simulink model "test_sim"  (R2020b)
settings: Solver=VariableStepAuto  StartTime=0.0  StopTime=10.0  RelTol=1e-3
libraries: fuzblock x1
settings Model: Creator=lima  LastModifiedBy=lima

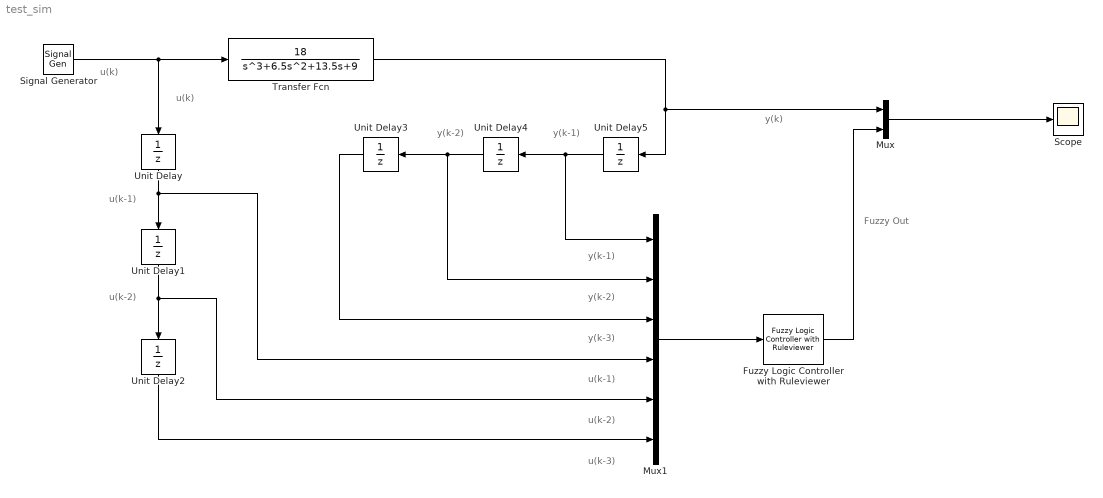
== system test_sim ==
  note: u(k)
  note: u(k-3)
  note: u(k-2)
  note: u(k-1)
  note: y(k-3)
  note: y(k-2)
  note: y(k-1)
  note: Fuzzy Out
  note: y(k)
  note: u(k)
  note: u(k-1)
  note: u(k-2)
  note: y(k-1)
  note: y(k-2)
  Fuzzy Logic Controller with Ruleviewer : fuzblock/Fuzzy Logic  Controller  with Ruleviewer  fismatrix=fis  Ts=2
  Mux : Mux  Inputs=2
  Mux1 : Mux  Inputs=6
  Scope : Scope
  Signal Generator : SignalGenerator  WaveForm=square  Units=rad/sec
  Transfer Fcn : TransferFcn  Numerator=[18]  Denominator=[1 6.5 13.5 9]
  Unit Delay{,1..5} (6 alike) : UnitDelay  SampleTime=-1  HasFrameUpgradeWarning=on
  wires:
  Unit Delay/1 -> Mux1/4, Unit Delay1/1
  Unit Delay1/1 -> Mux1/5, Unit Delay2/1
  Signal Generator/1 -> Transfer Fcn/1, Unit Delay/1
  Transfer Fcn/1 -> Unit Delay5/1, Mux/1
  Unit Delay5/1 -> Mux1/1, Unit Delay4/1
  Unit Delay4/1 -> Mux1/2, Unit Delay3/1
  Mux1/1 -> Fuzzy Logic Controller with Ruleviewer/1
  Fuzzy Logic Controller with Ruleviewer/1 -> Mux/2
  Mux/1 -> Scope/1
  Unit Delay3/1 -> Mux1/3
  Unit Delay2/1 -> Mux1/6
